simulink model "impl_dsgn"  (R2018b)
settings: Solver=VariableStepAuto  StartTime=1  StopTime=16  RelTol=1e-3
libraries: visiontextngfix x8, dspvision x5, visionsinks x4, library x3, visionstatistics x2, dspswit3 x1, visionanalysis x1
settings Model: Creator=dgaiero  LastModifiedBy=dgaiero

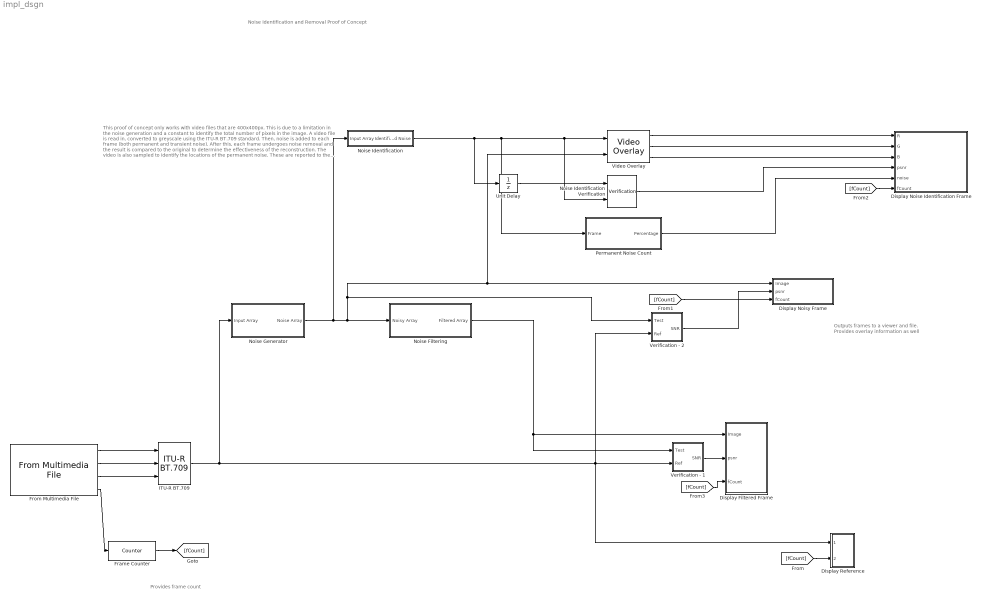
== system impl_dsgn ==
  note: Noise Identification and Removal Proof of Concept
  note: This proof of concept only works with video files that are 400x400px. This is due to a limitation in the noise generation and a constant to identify the total number of pixels in the image.
      |
      | A video file is read in, converted to greyscale using the ITU-R BT.709 standard. Then, noise is added to each frame (both permanent and transient noise).
      |
      | After this, each frame undergoes noise removal and the result is compared to the original to determine the effectiveness of the reconstruction.
      |
      | The video is also sampled to identify the locations of the permanent noise. These are reported to the user as well as identified how much of the frame is covered in permanent noise.
  note: Provides frame count
  note: Outputs frames to a viewer and file. Provides overlay information as well
  Display Filtered Frame : Subsystem
  Display Noise Identification Frame : Subsystem
  Display Noisy Frame : Subsystem
  Display Reference : Subsystem
  Frame Counter : dspswit3/Counter  Direction=Up  CountEvent=Free running  CounterSize=User defined  MaxCount=65535  InitialCount=1  Output=Count  HitValue=32  ResetInput=on  SamplesPerFrame=1  Ts=1/30  CntDtype=uint32  HitDtype=Logical
  From Multimedia File : dspvision/From Multimedia File  inputFilename=C:\Users\dgaiero\CY4Sym\quarter_1\cpe-446\finalPaper\design\Frames - conv.m4v  loop=on  numPlays=inf  outputStreams=Video only  videoDataType=single  audioDataType=int16  inheritSampleTime=on  userDefinedSampleTime=1/30  noAudioOutput=off  isIntensityVideo=off  fourcc=RGB  colorVideoFormat=Separate color signals  outputEOF=on  dataOrg=Column-major  audioFrameSize=1024  computeAudioFrameSize=off  outSamplingMode=Sample based
      settings: SourceProductBaseCode=VP
  ITU-R BT.709 : library/ITU-R BT.709  SystemSampleTime=-1
  Noise Filtering : Subsystem
  Noise Generator : Subsystem
  Noise Identification : Subsystem
  Noise Identification Verification : library/Verification  SystemSampleTime=-1
  Permanent Noise Count : Subsystem
  Unit Delay : UnitDelay  SampleTime=-1
  Verification - 1 : Subsystem
  Verification - 2 : Subsystem
  Video Overlay : library/Video Overlay  rChannelThreshold=0.7  gChannelThreshold=0.7  bChannelThreshold=0.7
  wires:
  From Multimedia File/1 -> ITU-R BT.709/1
  From Multimedia File/2 -> ITU-R BT.709/2
  From Multimedia File/3 -> ITU-R BT.709/3
  Noise Identification/1(Identified Noise) -> Permanent Noise Count/1(Frame), Noise Identification Verification/2, Video Overlay/1, Unit Delay/1
  Unit Delay/1 -> Noise Identification Verification/1
  From Multimedia File/4 -> Frame Counter/1
  Frame Counter/1 -> [fCount]
  Verification - 2/1(SNR) -> Display Noisy Frame/2(psnr)
  Verification - 1/1(SNR) -> Display Filtered Frame/2(psnr)
  Video Overlay/1 -> Display Noise Identification Frame/1(R)
  Video Overlay/2 -> Display Noise Identification Frame/2(G)
  Video Overlay/3 -> Display Noise Identification Frame/3(B)
  Noise Identification Verification/1 -> Display Noise Identification Frame/4(psnr)
  [fCount] -> Display Noise Identification Frame/6(fCount)
  [fCount] -> Display Noisy Frame/3(fCount)
  [fCount] -> Display Filtered Frame/3(fCount)
  [fCount] -> Display Reference/2(fCount)
  Permanent Noise Count/1(Percentage) -> Display Noise Identification Frame/5(noise)
  Noise Generator/1(Noise Array) -> Verification - 2/1(Test), Video Overlay/2, Display Noisy Frame/1(Image), Noise Filtering/1(Noisy Array), Noise Identification/1(Input Array)
  Noise Filtering/1(Filtered Array) -> Verification - 1/1(Test), Display Filtered Frame/1(Image)
  ITU-R BT.709/1 -> Verification - 2/2(Ref), Verification - 1/2(Ref), Display Reference/1(Image), Noise Generator/1(Input Array)

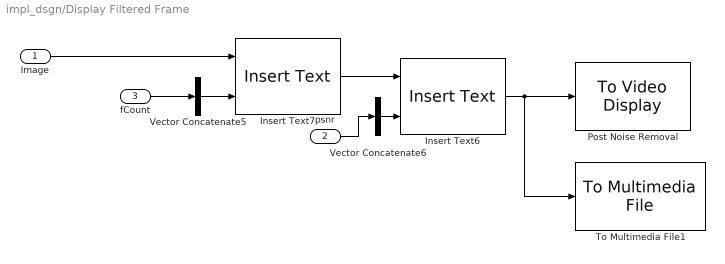
== system impl_dsgn/Display Filtered Frame ==
  Image : Inport
  psnr : Inport  Port=2
  fCount : Inport  Port=3
  Insert Text6 : visiontextngfix/Insert Text  inputType=Obsolete  theText='PSNR: %03.3f'  getTextLocFrom=Specify via dialog  textLoc=[1 12]  getTextColorFrom=Specify via dialog  textColor=[1 1 1]  getTextIntensityFrom=Specify via dialog  textIntensity=0  getTextOpacityFrom=Specify via dialog  textOpacity=1.0  dummyVar2=0  dummyVar3=0  dummyVar4=0  imagePorts=One multidimensional signal  isInputTransposed=off  fontFace=LucidaSansRegular  dummyVar1=0  blockFontSize=12  antiAliased=on
      settings: SourceProductName=Computer Vision System Toolbox  SourceProductBaseCode=VP
  Insert Text7 : visiontextngfix/Insert Text  inputType=Obsolete  theText='FRAME %04d'  getTextLocFrom=Specify via dialog  textLoc=[1 1]  getTextColorFrom=Specify via dialog  textColor=[1 1 1]  getTextIntensityFrom=Specify via dialog  textIntensity=0  getTextOpacityFrom=Specify via dialog  textOpacity=1.0  dummyVar2=0  dummyVar3=0  dummyVar4=0  imagePorts=One multidimensional signal  isInputTransposed=off  fontFace=LucidaSansRegular  dummyVar1=0  blockFontSize=12  antiAliased=on
      settings: SourceProductName=Computer Vision System Toolbox  SourceProductBaseCode=VP
  Post Noise Removal : visionsinks/To Video Display  windowSizeMode=Normal  openAtMdlStart=on  fullScreen=off  videoWindowX=-5801  videoWindowY=113  saveWindowSize=off  videoWindowWidth=1599  videoWindowHeight=1172  inputColorFormat=RGB  inputType=Obsolete  imagePorts=One multidimensional signal  OutputDevice=On-screen video monitor  dataOrg=Column-major  isWindowOpen=off
      settings: SourceProductName=Computer Vision System Toolbox
  To Multimedia File1 : dspvision/To Multimedia File  outputFilename=generated/postNR.avi  streamSelection=Video only  videoCompressor=None (uncompressed)  audioCompressor=None (uncompressed)  imagePorts=One multidimensional signal  fileType=AVI  audioDatatype=Determine from input data type  fourcc=RGB  videoQuality=75  mj2000CompFactor=10
      settings: SourceProductName=Computer Vision System Toolbox  SourceProductBaseCode=VP
  Vector Concatenate5 : Concatenate  NumInputs=1
  Vector Concatenate6 : Concatenate  NumInputs=1
  wires:
  Image/1 -> Insert Text7/1
  psnr/1 -> Vector Concatenate6/1
  Insert Text6/1 -> To Multimedia File1/1, Post Noise Removal/1
  Vector Concatenate5/1 -> Insert Text7/2
  Insert Text7/1 -> Insert Text6/1
  Vector Concatenate6/1 -> Insert Text6/2
  fCount/1 -> Vector Concatenate5/1

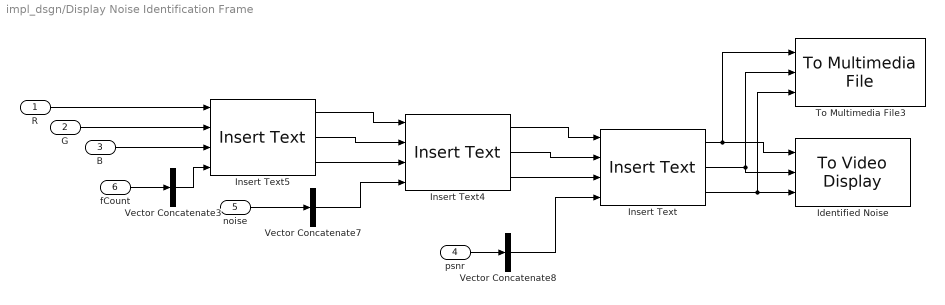
== system impl_dsgn/Display Noise Identification Frame ==
  R : Inport
  G : Inport  Port=2
  B : Inport  Port=3
  psnr : Inport  Port=4
  noise : Inport  Port=5
  fCount : Inport  Port=6
  Identified Noise : visionsinks/To Video Display  windowSizeMode=Normal  openAtMdlStart=on  fullScreen=off  videoWindowX=-5806  videoWindowY=1350  saveWindowSize=off  videoWindowWidth=1594  videoWindowHeight=1158  inputColorFormat=RGB  inputType=Obsolete  imagePorts=Separate color signals  OutputDevice=On-screen video monitor  dataOrg=Column-major  isWindowOpen=off
      settings: SourceProductName=Computer Vision System Toolbox
  Insert Text : visiontextngfix/Insert Text  inputType=Obsolete  theText='PSNR: %03.3f'  getTextLocFrom=Specify via dialog  textLoc=[1 24]  getTextColorFrom=Specify via dialog  textColor=[1 1 1]  getTextIntensityFrom=Specify via dialog  textIntensity=0  getTextOpacityFrom=Specify via dialog  textOpacity=1.0  dummyVar2=0  dummyVar3=0  dummyVar4=0  imagePorts=Separate color signals  isInputTransposed=off  fontFace=LucidaSansRegular  dummyVar1=0  blockFontSize=12  antiAliased=on
      settings: SourceProductName=Computer Vision System Toolbox  SourceProductBaseCode=VP
  Insert Text4 : visiontextngfix/Insert Text  inputType=Obsolete  theText='%% NOISE %2.3f%%'  getTextLocFrom=Specify via dialog  textLoc=[1 12]  getTextColorFrom=Specify via dialog  textColor=[1 1 1]  getTextIntensityFrom=Specify via dialog  textIntensity=0  getTextOpacityFrom=Specify via dialog  textOpacity=1.0  dummyVar2=0  dummyVar3=0  dummyVar4=0  imagePorts=Separate color signals  isInputTransposed=off  fontFace=LucidaSansRegular  dummyVar1=0  blockFontSize=12  antiAliased=on
      settings: SourceProductName=Computer Vision System Toolbox  SourceProductBaseCode=VP
  Insert Text5 : visiontextngfix/Insert Text  inputType=Obsolete  theText='FRAME %04d'  getTextLocFrom=Specify via dialog  textLoc=[1 1]  getTextColorFrom=Specify via dialog  textColor=[1 1 1]  getTextIntensityFrom=Specify via dialog  textIntensity=0  getTextOpacityFrom=Specify via dialog  textOpacity=1.0  dummyVar2=0  dummyVar3=0  dummyVar4=0  imagePorts=Separate color signals  isInputTransposed=off  fontFace=LucidaSansRegular  dummyVar1=0  blockFontSize=12  antiAliased=on
      settings: SourceProductName=Computer Vision System Toolbox  SourceProductBaseCode=VP
  To Multimedia File3 : dspvision/To Multimedia File  outputFilename=generated/noiseIdentification.avi  streamSelection=Video only  videoCompressor=None (uncompressed)  audioCompressor=None (uncompressed)  imagePorts=Separate color signals  fileType=AVI  audioDatatype=Determine from input data type  fourcc=RGB  videoQuality=75  mj2000CompFactor=10
      settings: SourceProductName=Computer Vision System Toolbox  SourceProductBaseCode=VP
  Vector Concatenate3 : Concatenate  NumInputs=1
  Vector Concatenate7 : Concatenate  NumInputs=1
  Vector Concatenate8 : Concatenate  NumInputs=1
  wires:
  Vector Concatenate3/1 -> Insert Text5/4
  Insert Text/1 -> To Multimedia File3/1, Identified Noise/1
  Insert Text5/3 -> Insert Text4/3
  Insert Text/3 -> To Multimedia File3/3, Identified Noise/3
  Insert Text/2 -> To Multimedia File3/2, Identified Noise/2
  Vector Concatenate7/1 -> Insert Text4/4
  B/1 -> Insert Text5/3
  psnr/1 -> Vector Concatenate8/1
  Insert Text5/2 -> Insert Text4/2
  Insert Text5/1 -> Insert Text4/1
  Insert Text4/2 -> Insert Text/2
  Insert Text4/1 -> Insert Text/1
  Vector Concatenate8/1 -> Insert Text/4
  fCount/1 -> Vector Concatenate3/1
  Insert Text4/3 -> Insert Text/3
  G/1 -> Insert Text5/2
  R/1 -> Insert Text5/1
  noise/1 -> Vector Concatenate7/1

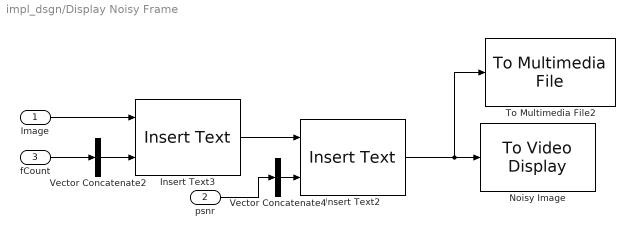
== system impl_dsgn/Display Noisy Frame ==
  Image : Inport
  psnr : Inport  Port=2
  fCount : Inport  Port=3
  Insert Text2 : visiontextngfix/Insert Text  inputType=Obsolete  theText='PSNR: %03.3f'  getTextLocFrom=Specify via dialog  textLoc=[1 12]  getTextColorFrom=Specify via dialog  textColor=[1 1 1]  getTextIntensityFrom=Specify via dialog  textIntensity=0  getTextOpacityFrom=Specify via dialog  textOpacity=1.0  dummyVar2=0  dummyVar3=0  dummyVar4=0  imagePorts=One multidimensional signal  isInputTransposed=off  fontFace=LucidaSansRegular  dummyVar1=0  blockFontSize=12  antiAliased=on
      settings: SourceProductName=Computer Vision System Toolbox  SourceProductBaseCode=VP
  Insert Text3 : visiontextngfix/Insert Text  inputType=Obsolete  theText='FRAME %04d'  getTextLocFrom=Specify via dialog  textLoc=[1 1]  getTextColorFrom=Specify via dialog  textColor=[1 1 1]  getTextIntensityFrom=Specify via dialog  textIntensity=0  getTextOpacityFrom=Specify via dialog  textOpacity=1.0  dummyVar2=0  dummyVar3=0  dummyVar4=0  imagePorts=One multidimensional signal  isInputTransposed=off  fontFace=LucidaSansRegular  dummyVar1=0  blockFontSize=12  antiAliased=on
      settings: SourceProductName=Computer Vision System Toolbox  SourceProductBaseCode=VP
  Noisy Image : visionsinks/To Video Display  windowSizeMode=Normal  openAtMdlStart=on  fullScreen=off  videoWindowX=-7401  videoWindowY=116  saveWindowSize=off  videoWindowWidth=1600  videoWindowHeight=1162  inputColorFormat=RGB  inputType=Obsolete  imagePorts=One multidimensional signal  OutputDevice=On-screen video monitor  dataOrg=Column-major  isWindowOpen=off
      settings: SourceProductName=Computer Vision System Toolbox
  To Multimedia File2 : dspvision/To Multimedia File  outputFilename=generated/noisyImage.avi  streamSelection=Video only  videoCompressor=None (uncompressed)  audioCompressor=None (uncompressed)  imagePorts=One multidimensional signal  fileType=AVI  audioDatatype=Determine from input data type  fourcc=RGB  videoQuality=75  mj2000CompFactor=10
      settings: SourceProductName=Computer Vision System Toolbox  SourceProductBaseCode=VP
  Vector Concatenate2 : Concatenate  NumInputs=1
  Vector Concatenate4 : Concatenate  NumInputs=1
  wires:
  Insert Text2/1 -> To Multimedia File2/1, Noisy Image/1
  Insert Text3/1 -> Insert Text2/1
  psnr/1 -> Vector Concatenate4/1
  Vector Concatenate4/1 -> Insert Text2/2
  Image/1 -> Insert Text3/1
  Vector Concatenate2/1 -> Insert Text3/2
  fCount/1 -> Vector Concatenate2/1

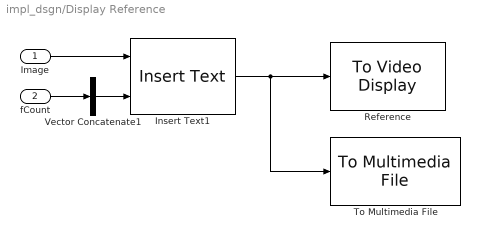
== system impl_dsgn/Display Reference ==
  Image : Inport
  fCount : Inport  Port=2
  Insert Text1 : visiontextngfix/Insert Text  inputType=Obsolete  theText='Frame %04d'  getTextLocFrom=Specify via dialog  textLoc=[1 1]  getTextColorFrom=Specify via dialog  textColor=[1 1 1]  getTextIntensityFrom=Specify via dialog  textIntensity=0  getTextOpacityFrom=Specify via dialog  textOpacity=1.0  dummyVar2=0  dummyVar3=0  dummyVar4=0  imagePorts=One multidimensional signal  isInputTransposed=off  fontFace=LucidaSansRegular  dummyVar1=0  blockFontSize=12  antiAliased=on
      settings: SourceProductName=Computer Vision System Toolbox  SourceProductBaseCode=VP
  Reference : visionsinks/To Video Display  windowSizeMode=Normal  openAtMdlStart=on  fullScreen=off  videoWindowX=-7409  videoWindowY=1345  saveWindowSize=off  videoWindowWidth=1603  videoWindowHeight=1153  inputColorFormat=RGB  inputType=Obsolete  imagePorts=One multidimensional signal  OutputDevice=On-screen video monitor  dataOrg=Column-major  isWindowOpen=off
      settings: SourceProductName=Computer Vision System Toolbox
  To Multimedia File : dspvision/To Multimedia File  outputFilename=generated/reference.avi  streamSelection=Video only  videoCompressor=None (uncompressed)  audioCompressor=None (uncompressed)  imagePorts=One multidimensional signal  fileType=AVI  audioDatatype=Determine from input data type  fourcc=RGB  videoQuality=75  mj2000CompFactor=10
      settings: SourceProductName=Computer Vision System Toolbox  SourceProductBaseCode=VP
  Vector Concatenate1 : Concatenate  NumInputs=1
  wires:
  Image/1 -> Insert Text1/1
  Insert Text1/1 -> To Multimedia File/1, Reference/1
  Vector Concatenate1/1 -> Insert Text1/2
  fCount/1 -> Vector Concatenate1/1

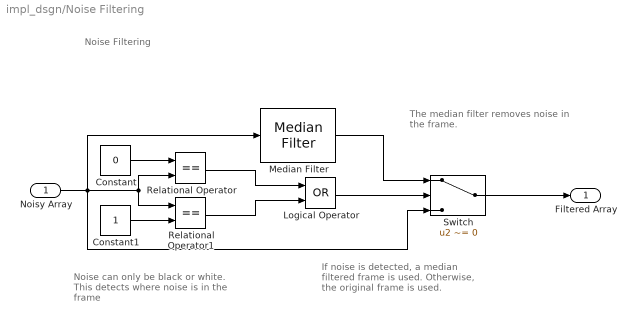
== system impl_dsgn/Noise Filtering ==
  note: Noise can only be black or white. This detects where noise is in the frame
  note: Noise Filtering
  note: If noise is detected, a median filtered frame is used. Otherwise, the original frame is used.
  note: The median filter removes noise in the frame.
  Noisy Array : Inport
  Constant : Constant  Value=0  SampleTime=-1
  Constant1 : Constant  SampleTime=-1
  Logical Operator : Logic  Operator=OR  AllPortsSameDT=off  OutDataTypeStr=boolean
  Median Filter : visionanalysis/Median Filter  nghbood=[3 3]  outSize=Same as input port I  padType=Symmetric  padSrc=Specify via dialog  padVal=0  roundingMode=Floor  overflowMode=off
      settings: SourceProductName=Computer Vision System Toolbox  SourceProductBaseCode=VP
  Relational Operator : RelationalOperator  Operator===  OutDataTypeStr=boolean  RndMeth=Nearest
  Relational Operator1 : RelationalOperator  Operator===  OutDataTypeStr=boolean  RndMeth=Nearest
  Switch : Switch  Criteria=u2 ~= 0
  Filtered Array : Outport
  wires:
  Logical Operator/1 -> Switch/2
  Noisy Array/1 -> Switch/3, Median Filter/1, Relational Operator/2, Relational Operator1/1
  Relational Operator/1 -> Logical Operator/1
  Relational Operator1/1 -> Logical Operator/2
  Constant/1 -> Relational Operator/1
  Constant1/1 -> Relational Operator1/2
  Switch/1 -> Filtered Array/1
  Median Filter/1 -> Switch/1

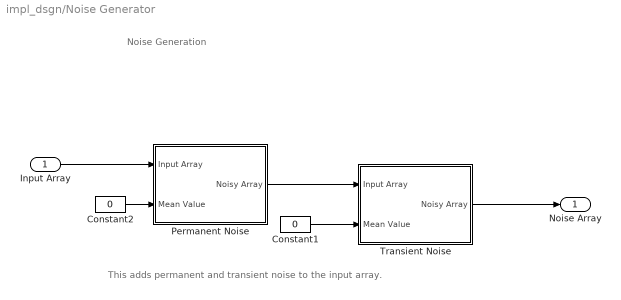
== system impl_dsgn/Noise Generator ==
  note: This adds permanent and transient noise to the input array.
  note: Noise Generation
  Input Array : Inport
  Constant1 : Constant  Value=0  SampleTime=-1
  Constant2 : Constant  Value=0  SampleTime=-1
  Permanent Noise : Subsystem  mask{Gain=50}
      mask prompts: Gain "Simulink:blkprm_prompts:GainGain"
      mask TypeOptions Gain: Oversaturation Control/Gain
      mask DialogControl Gain Prompt: Gain:
  Transient Noise : Subsystem  mask{Gain=100}
      mask prompts: Gain "Simulink:blkprm_prompts:GainGain"
      mask TypeOptions Gain: Oversaturation Control/Gain
      mask DialogControl Gain Prompt: Gain:
  Noise Array : Outport
  wires:
  Input Array/1 -> Permanent Noise/1(Input Array)
  Constant2/1 -> Permanent Noise/2(Mean Value)
  Constant1/1 -> Transient Noise/2(Mean Value)
  Permanent Noise/1(Noisy Array) -> Transient Noise/1(Input Array)
  Transient Noise/1(Noisy Array) -> Noise Array/1

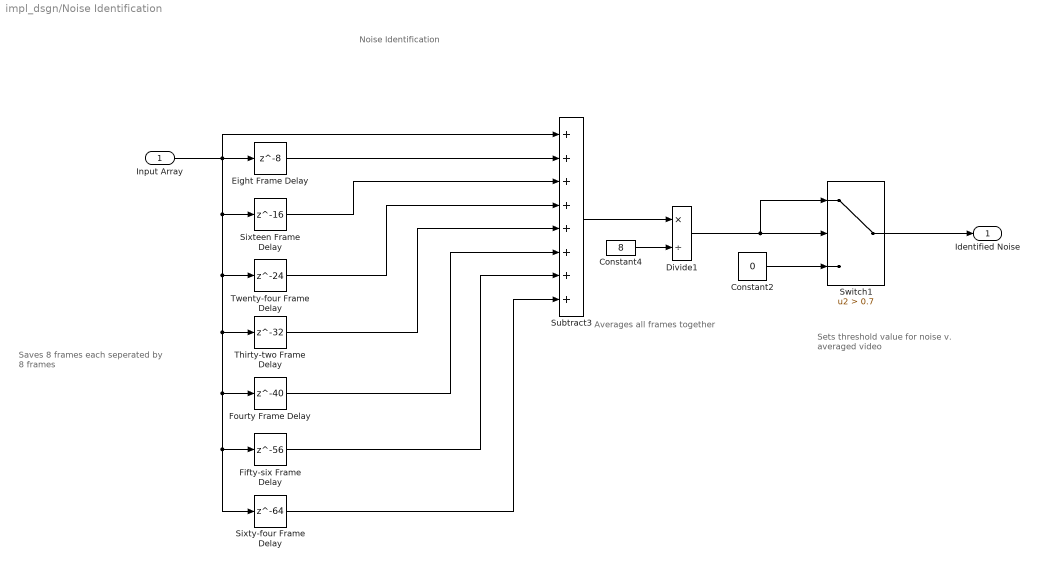
== system impl_dsgn/Noise Identification ==
  note: Saves 8 frames each seperated by 8 frames
  note: Noise Identification
  note: Averages all frames together
  note: Sets threshold value for noise v. averaged video
  Input Array : Inport
  Constant2 : Constant  Value=0  SampleTime=-1
  Constant4 : Constant  Value=8  SampleTime=-1
  Divide1 : Product  Inputs=*/  SaturateOnIntegerOverflow=on  RndMeth=Zero
  Eight Frame Delay : Delay  DelayLength=8
  Fifty-six Frame Delay : Delay  DelayLength=56
  Fourty Frame Delay : Delay  DelayLength=40
  Sixteen Frame Delay : Delay  DelayLength=16
  Sixty-four Frame Delay : Delay  DelayLength=64
  Subtract3 : Sum  Inputs=++++++++
  Switch1 : Switch  Criteria=u2 > Threshold  Threshold=0.7
  Thirty-two Frame Delay : Delay  DelayLength=32
  Twenty-four Frame Delay : Delay  DelayLength=24
  Identified Noise : Outport
  wires:
  Input Array/1 -> Subtract3/1, Fifty-six Frame Delay/1, Sixty-four Frame Delay/1, Fourty Frame Delay/1, Thirty-two Frame Delay/1, Twenty-four Frame Delay/1, Sixteen Frame Delay/1, Eight Frame Delay/1
  Constant2/1 -> Switch1/3
  Eight Frame Delay/1 -> Subtract3/2
  Sixteen Frame Delay/1 -> Subtract3/3
  Twenty-four Frame Delay/1 -> Subtract3/4
  Thirty-two Frame Delay/1 -> Subtract3/5
  Fourty Frame Delay/1 -> Subtract3/6
  Fifty-six Frame Delay/1 -> Subtract3/7
  Sixty-four Frame Delay/1 -> Subtract3/8
  Subtract3/1 -> Divide1/1
  Constant4/1 -> Divide1/2
  Divide1/1 -> Switch1/1, Switch1/2
  Switch1/1 -> Identified Noise/1

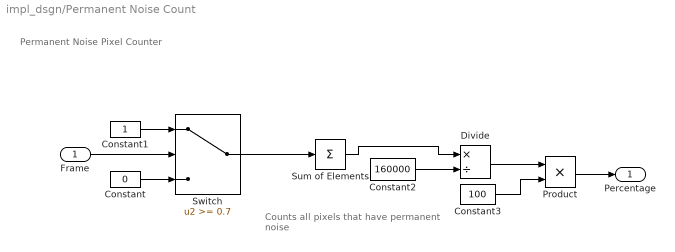
== system impl_dsgn/Permanent Noise Count ==
  note: Counts all pixels that have permanent noise
  note: Permanent Noise Pixel Counter
  Frame : Inport
  Constant : Constant  Value=0  SampleTime=-1
  Constant1 : Constant  SampleTime=-1
  Constant2 : Constant  Value=160000  SampleTime=-1
  Constant3 : Constant  Value=100  SampleTime=-1
  Divide : Product  Inputs=*/  SaturateOnIntegerOverflow=on  RndMeth=Zero
  Product : Product
  Sum of Elements : Sum  Inputs=+
  Switch : Switch  Threshold=0.7
  Percentage : Outport
  wires:
  Constant/1 -> Switch/3
  Frame/1 -> Switch/2
  Divide/1 -> Product/1
  Constant1/1 -> Switch/1
  Switch/1 -> Sum of Elements/1
  Sum of Elements/1 -> Divide/1
  Product/1 -> Percentage/1
  Constant3/1 -> Product/2
  Constant2/1 -> Divide/2

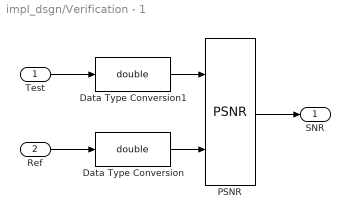
== system impl_dsgn/Verification - 1 ==
  Test : Inport
  Ref : Inport  Port=2
  Data Type Conversion : DataTypeConversion  OutDataTypeStr=double
  Data Type Conversion1 : DataTypeConversion  OutDataTypeStr=double
  PSNR : visionstatistics/PSNR
      settings: SourceProductName=Computer Vision System Toolbox  SourceProductBaseCode=VP
  SNR : Outport
  wires:
  Data Type Conversion/1 -> PSNR/2
  PSNR/1 -> SNR/1
  Test/1 -> Data Type Conversion1/1
  Ref/1 -> Data Type Conversion/1
  Data Type Conversion1/1 -> PSNR/1

== system impl_dsgn/Verification - 2 ==
  Test : Inport
  Ref : Inport  Port=2
  Data Type Conversion : DataTypeConversion  OutDataTypeStr=double
  Data Type Conversion1 : DataTypeConversion  OutDataTypeStr=double
  PSNR : visionstatistics/PSNR
      settings: SourceProductName=Computer Vision System Toolbox  SourceProductBaseCode=VP
  SNR : Outport
  wires:
  Data Type Conversion/1 -> PSNR/2
  PSNR/1 -> SNR/1
  Test/1 -> Data Type Conversion1/1
  Ref/1 -> Data Type Conversion/1
  Data Type Conversion1/1 -> PSNR/1

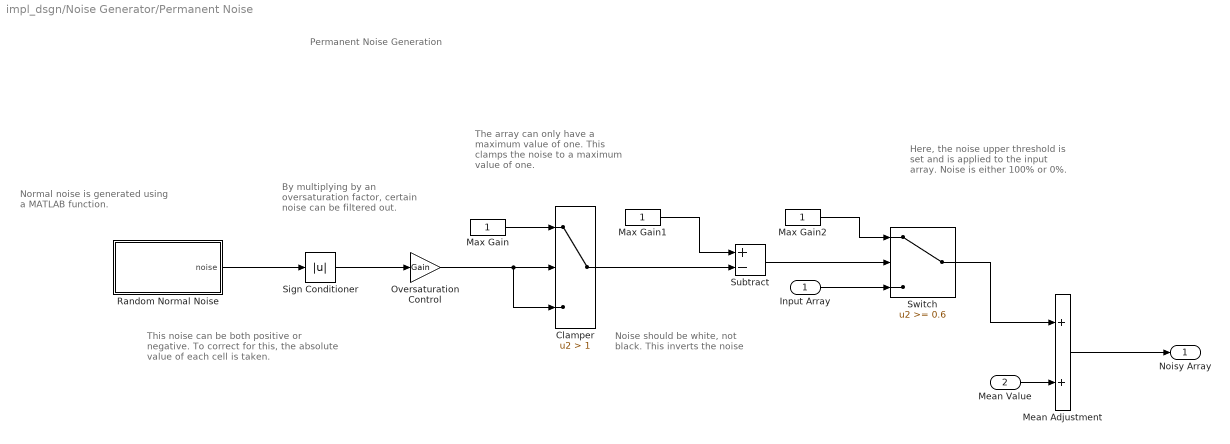
== system impl_dsgn/Noise Generator/Permanent Noise ==
  note: Permanent Noise Generation
  note: Normal noise is generated using a MATLAB function.
  note: This noise can be both positive or negative. To correct for this, the absolute value of each cell is taken.
  note: By multiplying by an oversaturation factor, certain noise can be filtered out.
  note: The array can only have a maximum value of one. This clamps the noise to a maximum value of one.
  note: Noise should be white, not black. This inverts the noise
  note: Here, the noise upper threshold is set and is applied to the input array. Noise is either 100% or 0%.
  Input Array : Inport
  Mean Value : Inport  Port=2
  Clamper : Switch  Criteria=u2 > Threshold  Threshold=1
  Max Gain : Constant  SampleTime=-1
  Max Gain1 : Constant  SampleTime=-1
  Max Gain2 : Constant  SampleTime=-1
  Mean Adjustment : Sum
  Oversaturation Control : Gain  Gain=Gain
  Random Normal Noise : MATLAB Function  TreatAsAtomicUnit=on
  Sign Conditioner : Abs
  Subtract : Sum  Inputs=+-
  Switch : Switch  Threshold=0.6
  Noisy Array : Outport
  wires:
  Switch/1 -> Mean Adjustment/1
  Mean Value/1 -> Mean Adjustment/2
  Random Normal Noise/1(noise) -> Sign Conditioner/1
  Sign Conditioner/1 -> Oversaturation Control/1
  Clamper/1 -> Subtract/2
  Max Gain/1 -> Clamper/1
  Mean Adjustment/1 -> Noisy Array/1
  Oversaturation Control/1 -> Clamper/3, Clamper/2
  Max Gain1/1 -> Subtract/1
  Subtract/1 -> Switch/2
  Input Array/1 -> Switch/3
  Max Gain2/1 -> Switch/1

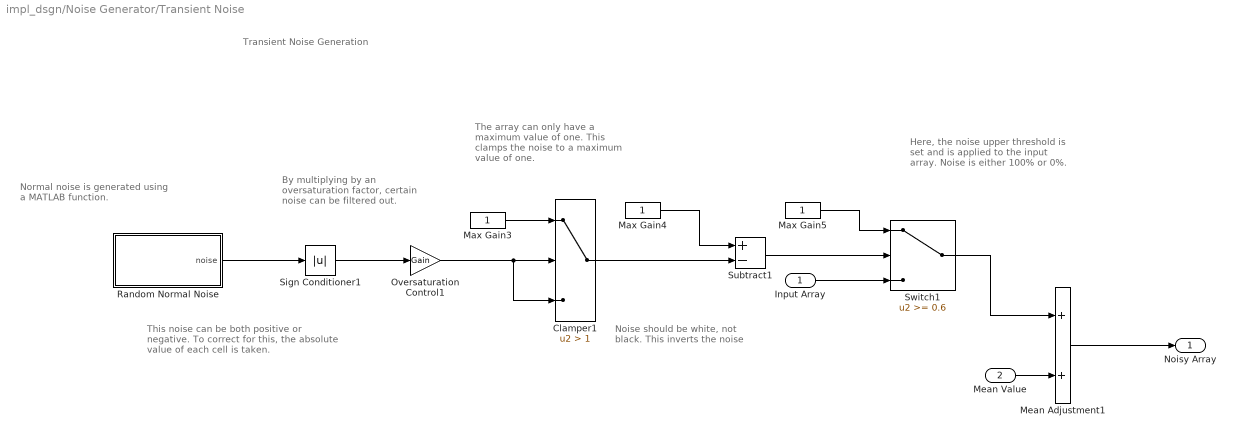
== system impl_dsgn/Noise Generator/Transient Noise ==
  note: By multiplying by an oversaturation factor, certain noise can be filtered out.
  note: Transient Noise Generation
  note: Here, the noise upper threshold is set and is applied to the input array. Noise is either 100% or 0%.
  note: Normal noise is generated using a MATLAB function.
  note: This noise can be both positive or negative. To correct for this, the absolute value of each cell is taken.
  note: Noise should be white, not black. This inverts the noise
  note: The array can only have a maximum value of one. This clamps the noise to a maximum value of one.
  Input Array : Inport
  Mean Value : Inport  Port=2
  Clamper1 : Switch  Criteria=u2 > Threshold  Threshold=1
  Max Gain3 : Constant  SampleTime=-1
  Max Gain4 : Constant  SampleTime=-1
  Max Gain5 : Constant  SampleTime=-1
  Mean Adjustment1 : Sum
  Oversaturation Control1 : Gain  Gain=Gain
  Random Normal Noise : MATLAB Function  TreatAsAtomicUnit=on
  Sign Conditioner1 : Abs
  Subtract1 : Sum  Inputs=+-
  Switch1 : Switch  Threshold=0.6
  Noisy Array : Outport
  wires:
  Clamper1/1 -> Subtract1/2
  Max Gain3/1 -> Clamper1/1
  Mean Value/1 -> Mean Adjustment1/2
  Max Gain4/1 -> Subtract1/1
  Sign Conditioner1/1 -> Oversaturation Control1/1
  Max Gain5/1 -> Switch1/1
  Mean Adjustment1/1 -> Noisy Array/1
  Subtract1/1 -> Switch1/2
  Switch1/1 -> Mean Adjustment1/1
  Random Normal Noise/1(noise) -> Sign Conditioner1/1
  Input Array/1 -> Switch1/3
  Oversaturation Control1/1 -> Clamper1/3, Clamper1/2

== matlab function impl_dsgn/Noise Generator/Permanent Noise/Random Normal Noise ==
  data: noise output size=[400 400]
function noise = fcn()
    rng(100);
    noise = randn(400);

== matlab function impl_dsgn/Noise Generator/Transient Noise/Random Normal Noise ==
  data: noise output size=[400 400]
function noise = fcn()
    rng('shuffle');
    noise = randn(400);
